simulink model "first"  (R2020a)
settings: Solver=VariableStepAuto  StartTime=0.0  StopTime=10.0  RelTol=1e-3
settings Model: Creator=Admin  LastModifiedBy=Admin

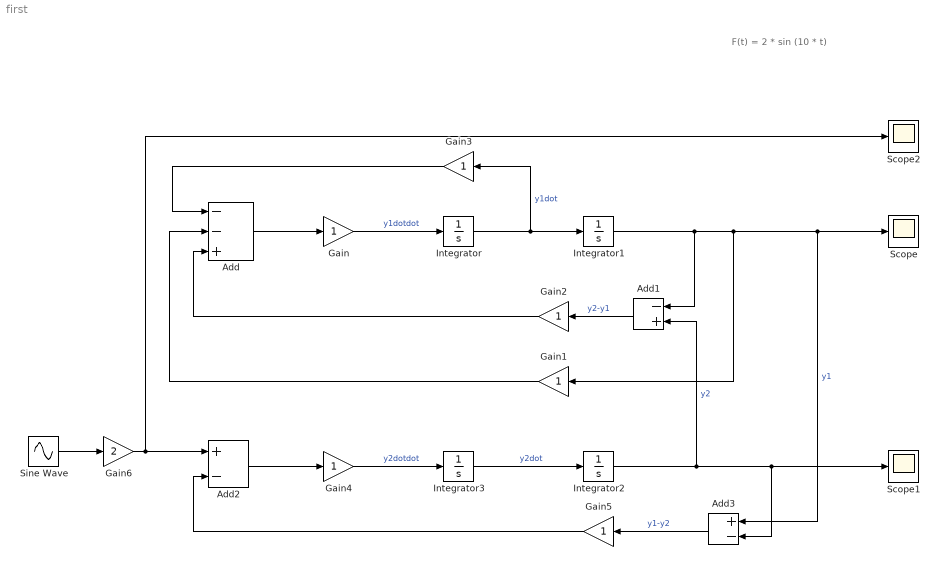
== system first ==
  note: F(t) = 2 * sin (10 * t)
  Add : Sum  Inputs=--+
  Add1 : Sum  Inputs=-+
  Add2 : Sum  Inputs=+-
  Add3 : Sum  Inputs=+-
  Gain{,1..5} (6 alike) : Gain
  Gain6 : Gain  Gain=2
  Integrator{,1..3} (4 alike) : Integrator
  Scope : Scope
  Scope1 : Scope
  Scope2 : Scope
  Sine Wave : Sin  SampleTime=0
  wires:
  Add/1 -> Gain/1
  Integrator/1 -> Gain3/1, Integrator1/1  "y1dot"
  Gain/1 -> Integrator/1  "y1dotdot"
  Integrator1/1 -> Add1/1, Gain1/1, Add3/1, Scope/1  "y1"
  Integrator2/1 -> Add1/2, Add3/2, Scope1/1  "y2"
  Integrator3/1 -> Integrator2/1  "y2dot"
  Add1/1 -> Gain2/1  "y2-y1"
  Gain2/1 -> Add/3
  Gain1/1 -> Add/2
  Gain3/1 -> Add/1
  Gain4/1 -> Integrator3/1  "y2dotdot"
  Add2/1 -> Gain4/1
  Add3/1 -> Gain5/1  "y1-y2"
  Gain5/1 -> Add2/2
  Sine Wave/1 -> Gain6/1
  Gain6/1 -> Scope2/1, Add2/1
